simulink model "closed_loop_try"  (R2023b)
settings: Solver=VariableStepAuto  StartTime=0.0  StopTime=10.0  RelTol=1e-3
values from neighbouring files (symbols this model uses):
  N = 20    [car_PDM_ocp.m]    (also in closed_loop.m; main.m = 40; main_velocity_simple.m = 100; simple_test.m = 500)
  Ts = 0.01    [car_PDM_ocp.m]    (also in closed_loop.m; main.m; main_velocity_simple.m; simple_test.m = 0.25)
  V0 = par.V0    [car_PDM_ocp.m]    (also in main_velocity_simple.m)
undefined symbols (not defined in the file or in its folder): par
settings Model: Creator=maart  LastModifiedBy=maart

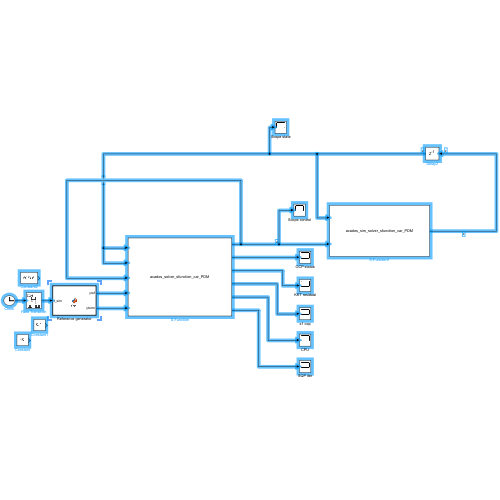
[thumbnail: Simulink's stored preview of the top-level diagram]
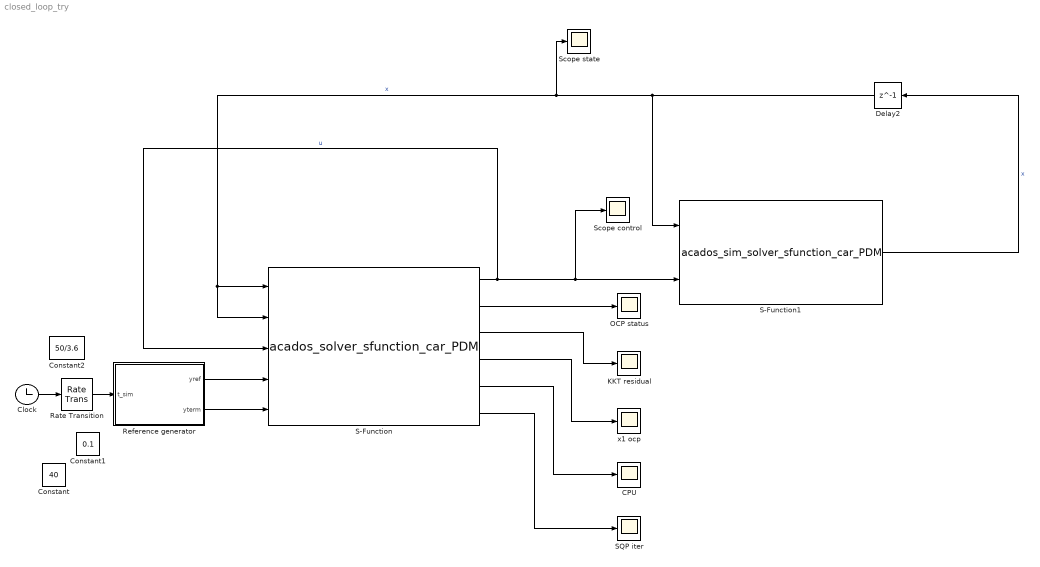
== system closed_loop_try ==
  CPU : Scope
      settings: Description=status
  Clock : Clock
  Constant : Constant  Value=40
  Constant1 : Constant  Value=0.1
  Constant2 : Constant  Value=50/3.6
  Delay2 : Delay  DelayLength=1  InitialCondition=[par.V0,0,0,0,0,0,0]
  KKT residual : Scope
      settings: Description=status
  OCP status : Scope
      settings: Description=status
  Rate Transition : RateTransition
  Reference generator : MATLAB Function  TreatAsAtomicUnit=on
  S-Function : S-Function  FunctionName=acados_solver_sfunction_car_PDM  SFunctionDeploymentMode=off  EnableBusSupport=off
  S-Function1 : S-Function  FunctionName=acados_sim_solver_sfunction_car_PDM  SFunctionDeploymentMode=off  EnableBusSupport=off
  SQP iter : Scope
      settings: Description=status
  Scope control : Scope
  Scope state : Scope
  x1 ocp : Scope
      settings: Description=status
  wires:
  Clock/1 -> Rate Transition/1
  Reference generator/1(yref) -> S-Function/4
  Reference generator/2(yterm) -> S-Function/5
  S-Function/4 -> x1 ocp/1
  S-Function/6 -> SQP iter/1
  S-Function/5 -> CPU/1
  S-Function/2 -> OCP status/1
  S-Function/3 -> KKT residual/1
  S-Function/1 -> Scope control/1, S-Function1/2, S-Function/3  "u"
  S-Function1/1 -> Delay2/1  "x"
  Delay2/1 -> S-Function1/1, Scope state/1, S-Function/1, S-Function/2  "x"
  Rate Transition/1 -> Reference generator/1(t_sim)

== matlab function closed_loop_try/Reference generator ==
  data: yref output; t_sim input size=1; yterm output; V0 parameter size=1; N parameter size=1; Ts parameter size=1
function [yref,yterm] = fcn(t_sim, V0, N, Ts)

    % t = t_sim + Ts*(1:N);
    % 
    % [~, Xp_ref, Yp_ref] = reference_corner(V0, t);
    % 
    % if length(Xp_ref) == 1
    %     Xp_ref = repmat(Xp_ref,1,N); 
    % end
    % 
    % if length(Yp_ref) == 1
    %     Yp_ref = repmat(Yp_ref,1,N);
    % end
    % 
    % arrayV0 = repmat(V0,1,N-1);
    % array0 = zeros(5,N-1);
    % 
    % yref = zeros(1,312);
    % yterm = zeros(1,7);
    % 
    % yref = reshape([arrayV0;Xp_ref(1:end-1);Yp_ref(1:end-1);array0],1,[]);
    % 
    % yterm = [V0;Xp_ref(end);Yp_ref(end);array0(:,1)];

    yref = zeros(1,8*(N-1));

    for i=1:N-1
        t = t_sim + Ts*i;

        [~, Xp_ref, Yp_ref] = reference_corner(V0, t);

        yref(1+8*(i-1):8*(i-1)+8) = [V0;Xp_ref;Yp_ref;zeros(5,1)];

    end

    [~, Xp_ref, Yp_ref] = reference_corner(V0, (t_sim + Ts*N));

    yterm = [V0;Xp_ref;Yp_ref;zeros(4,1)];
